simulink model "asbGravWPrec"  (R2023a)
settings: Solver=VariableStepDiscrete  StartTime=0.0  StopTime=10.0  MaxStep=0.2  RelTol=1e-3  EnableMultiTasking=on
libraries: aerolibgravity2 x2, aerolibtransform2 x1, aerolibconvert2 x1, simulink x1
Description:
  | Gravity Models with Precessing Reference Frame
  | 
  | This model shows how to implement various gravity models with precessing reference frames
  | using Aerospace Blockset(TM) blocks.  The Aerospace Blockset blocks are shown in red.
settings Model: Creator=The MathWorks, Inc.  LastModifiedBy=The MathWorks, Inc.
settings SolverCC: AlgebraicLoopSolver=TrustRegion
settings DataIOCC: LimitDataPoints=on  SaveFormat=Array  ReturnWorkspaceOutputs=off
settings OptimizationCC: ReuseModelBlockBuffer=off  ExpressionDepthLimit=2147483647  LifeSpan=inf
settings DebuggingCC: SolverPrmCheckMsg=warning  FcnCallInpInsideContextMsg=warning  UnconnectedInputMsg=warning  UnconnectedOutputMsg=warning  UnconnectedLineMsg=warning  UniqueDataStoreMsg=error  StateNameClashWarn=warning  StrictBusMsg=ErrorOnBusTreatedAsVector  SFUnexpectedBacktrackingDiag=warning  SFNoUnconditionalDefaultTransitionDiag=warning  SFExecutionAtInitializationDiag=none  ArithmeticOperatorsInVariantConditions=warning
settings HardwareCC: ProdBitPerPointer=32  ProdBitPerSizeT=32  ProdBitPerPtrDiffT=32  ProdLargestAtomicFloat=None  ProdIntDivRoundTo=Undefined  ProdEndianess=Unspecified  ProdWordSize=32  ProdHWDeviceType=32-bit Generic
settings ModelReferenceCC: EnableRefExpFcnMdlSchedulingChecks=on  PropagateSignalLabelsOutOfModel=off
settings SFSimCC: SimUseLocalCustomCode=off  CustomCodeUndefinedFunction=UseInterfaceOnly
settings RTWCC: RTWUseLocalCustomCode=off
settings CodeAppCC: StateflowObjectComments=on
settings GRTTargetCC: TargetLangStandard=C89/C90 (ANSI)  CombineOutputUpdateFcns=off  GRTInterface=on
settings ConfigComp: CovMetricSettings=dw  CovSaveCumulativeToWorkspaceVar=on  CovSaveSingleToWorkspaceVar=on  CovExternalEMLEnable=off

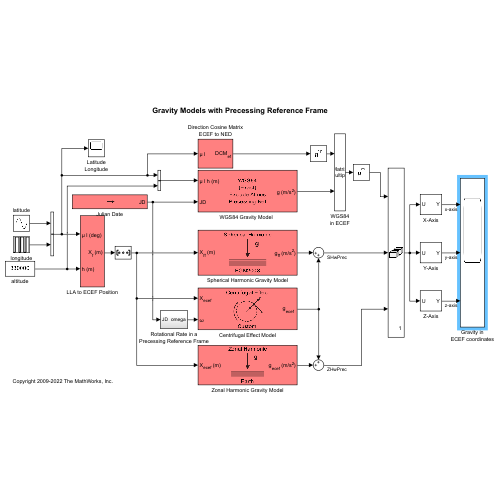
[thumbnail: Simulink's stored preview of the top-level diagram]
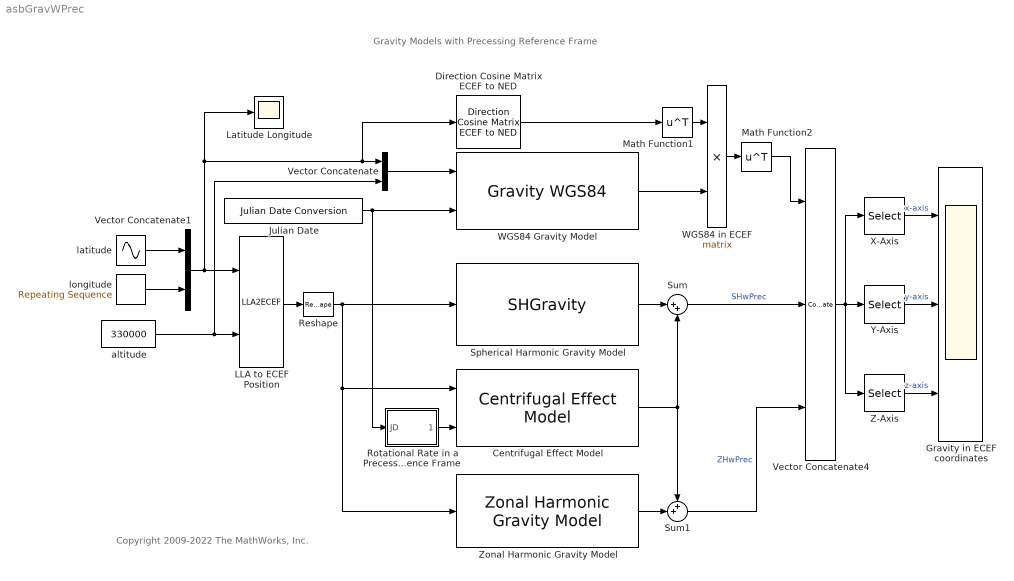
== system asbGravWPrec ==
  note: Copyright 2009-2022 The MathWorks, Inc.
  note: Gravity Models with Precessing Reference Frame
  Centrifugal Effect Model : aerolibgravity2/Centrifugal Effect Model  ptype=Custom  omega=7.2921150e-005  rate_loc=on
  Direction Cosine Matrix ECEF to NED : aerolibtransform2/Direction Cosine Matrix ECEF to NED
  Gravity in ECEF coordinates : Scope  NumInputPorts=3
  Julian Date : aerolibconvert2/Julian Date Conversion  year=2004  month=October  day=10  hour=12  min=21  sec=0  modflag=off  deltaT=None  errorflag=Error
  LLA to ECEF Position : LLA2ECEF  R=6378137
  Latitude Longitude : Scope
  Math Function1 : Math  Operator=transpose  SignedPower=on
  Math Function2 : Math  Operator=transpose  SignedPower=on
  Reshape : Reshape  OutputDimensionality=Row vector (2-D)
  Rotational Rate in a Precessing Reference Frame : Subsystem
  Spherical Harmonic Gravity Model : SHGravity  datafile='aerogmm2b'
  Sum : Sum  Inputs=|++
  Sum1 : Sum  Inputs=++|
  Vector Concatenate : Concatenate
  Vector Concatenate1 : Concatenate
  Vector Concatenate4 : Concatenate  NumInputs=3  Mode=Multidimensional array
  WGS84 in ECEF : Product  Multiplication=Matrix(*)  RndMeth=Zero
  "WGS84 Gravity Model  " : GravityWGS84  model=WGS84 Exact  jd_loc=on  no_centrifugal=off  action=None
  X-Axis : Selector  NumberOfDimensions=2  IndexMode=Zero-based  InputPortWidth=3  IndexOptions=Index vector (dialog),Index vector (dialog)  Indices=[0 1 2],0  OutputSizes=1,1
  Y-Axis : Selector  NumberOfDimensions=2  IndexMode=Zero-based  InputPortWidth=3  IndexOptions=Index vector (dialog),Index vector (dialog)  Indices=[0 1 2],1  OutputSizes=1,1
  Z-Axis : Selector  NumberOfDimensions=2  IndexMode=Zero-based  InputPortWidth=3  IndexOptions=Index vector (dialog),Index vector (dialog)  Indices=[0 1 2],2  OutputSizes=1,1
  Zonal Harmonic Gravity Model : aerolibgravity2/Zonal Harmonic Gravity Model  units=Metric (MKS)  degree=4  action=Warning  ptype=Earth  R=6378136.3  GM=398600441500000  jvalue=[1.0826269e-03 -2.5323000e-06 -1.6204000e-06]
  altitude : Constant  Value=330000
  latitude : Sin  Amplitude=[90 ]  Frequency=pi/5  SampleTime=0
  longitude : simulink/Sources/Repeating Sequence  rep_seq_t=[ 0 2.5 2.5+eps(2.5) 7.5]  rep_seq_y=[ 0 0 180+0*eps(2.5) 180]
  wires:
  Spherical Harmonic Gravity Model/1 -> Sum/1
  Centrifugal Effect Model/1 -> Sum/2, Sum1/1
  Zonal Harmonic Gravity Model/1 -> Sum1/2
  Vector Concatenate1/1 -> LLA to ECEF Position/1, Vector Concatenate/1, Direction Cosine Matrix ECEF to NED/1, Latitude Longitude/1
  altitude/1 -> Vector Concatenate/2, LLA to ECEF Position/2
  LLA to ECEF Position/1 -> Reshape/1
  Vector Concatenate/1 -> "WGS84 Gravity Model  "/1
  Reshape/1 -> Zonal Harmonic Gravity Model/1, Centrifugal Effect Model/1, Spherical Harmonic Gravity Model/1
  Rotational Rate in a Precessing Reference Frame/1(omega) -> Centrifugal Effect Model/2
  Julian Date/1 -> "WGS84 Gravity Model  "/2, Rotational Rate in a Precessing Reference Frame/1(JD)
  "WGS84 Gravity Model  "/1 -> WGS84 in ECEF/2
  Direction Cosine Matrix ECEF to NED/1 -> Math Function1/1
  Math Function1/1 -> WGS84 in ECEF/1
  X-Axis/1 -> Gravity in ECEF coordinates/1  "x-axis"
  Y-Axis/1 -> Gravity in ECEF coordinates/2  "y-axis"
  Z-Axis/1 -> Gravity in ECEF coordinates/3  "z-axis"
  WGS84 in ECEF/1 -> Math Function2/1
  Math Function2/1 -> Vector Concatenate4/1
  Sum/1 -> Vector Concatenate4/2  "SHwPrec"
  Sum1/1 -> Vector Concatenate4/3  "ZHwPrec"
  Vector Concatenate4/1 -> Y-Axis/1, X-Axis/1, Z-Axis/1
  longitude/1 -> Vector Concatenate1/2
  latitude/1 -> Vector Concatenate1/1

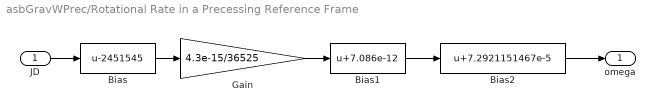
== system asbGravWPrec/Rotational Rate in a Precessing Reference Frame ==
  JD : Inport
  Bias : Bias  Bias=-2451545  SaturateOnIntegerOverflow=off
  Bias1 : Bias  Bias=7.086e-12  SaturateOnIntegerOverflow=off
  Bias2 : Bias  Bias=7.2921151467e-5  SaturateOnIntegerOverflow=off
  Gain : Gain  Gain=4.3e-15/36525
  omega : Outport  VectorParamsAs1DForOutWhenUnconnected=off
  wires:
  JD/1 -> Bias/1
  Bias/1 -> Gain/1
  Gain/1 -> Bias1/1
  Bias1/1 -> Bias2/1
  Bias2/1 -> omega/1
